simulink model "LAB1_REDES_CONV"  (R2024b)
settings: Solver=VariableStepAuto  StartTime=0.0  StopTime=inf  RelTol=1e-3
undefined symbols (not defined in the file): QAM
libraries: simulink_extras x4, commdigbbndam3 x2, dspvision x1, simulink x1, commrandsrc3 x1
settings Model: Creator=ASUS  LastModifiedBy=ASUS

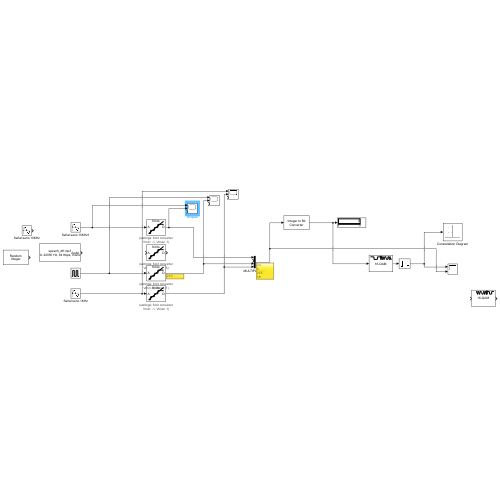
[thumbnail: Simulink's stored preview of the top-level diagram]
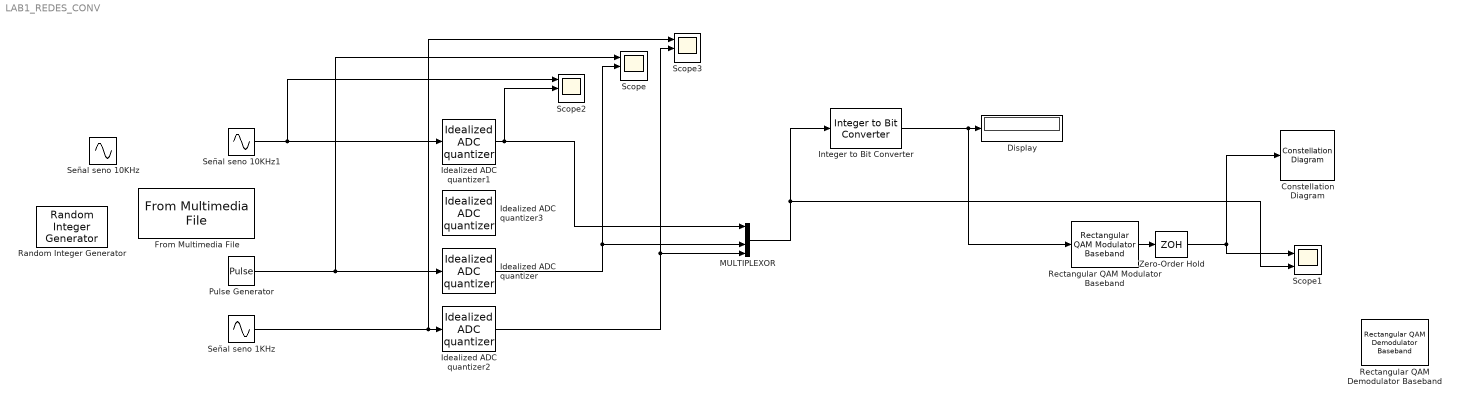
== system LAB1_REDES_CONV ==
  Constellation Diagram : ConstellationDiagram  WindowPosition=[88.000000,123.000000,600.000000,600.000000,]  Visible=on  ScopeFrameLocation=window  ReferenceConstellation=16-QAM  XLimits=[-1.24,1.38]  YLimits=[-1.15,1.28]  ShowReferenceConstellation=off  MeasurementInterval=All displays  DefaultConfigurationName=comm.scopes.ConstellationDiagramBlockCfg
  Display : Display
  From Multimedia File : dspvision/From Multimedia File  inputFilename=speech_dft.mp3  readRange=[1 Inf]  loop=on  numPlays=inf  outputStreams=Audio only  videoDataType=single  audioDataType=double  inheritSampleTime=on  userDefinedSampleTime=1/30  noAudioOutput=off  isIntensityVideo=off  fourcc=RGB  colorVideoFormat=Separate color signals  outputEOF=off  dataOrg=Column-major  audioFrameSize=1024  computeAudioFrameSize=off  outSamplingMode=Sample based
      settings: LibrarySourceBlock=audiosources/From Multimedia File
  Idealized ADC quantizer : simulink_extras/Additional Discrete/Idealized ADC quantizer  NumberOfConverterBits=8  Vmin=0  Vmax=1  OutputDataType=uint8  OutputNegativeValues=on
  Idealized ADC quantizer1 : simulink_extras/Additional Discrete/Idealized ADC quantizer  NumberOfConverterBits=8  Vmin=-1  Vmax=1  OutputDataType=uint8  OutputNegativeValues=off
  Idealized ADC quantizer2 : simulink_extras/Additional Discrete/Idealized ADC quantizer  NumberOfConverterBits=8  Vmin=-1  Vmax=1  OutputDataType=uint8  OutputNegativeValues=off
  Idealized ADC quantizer3 : simulink_extras/Additional Discrete/Idealized ADC quantizer  NumberOfConverterBits=8  Vmin=0  Vmax=5  OutputDataType=uint8  OutputNegativeValues=on
  Integer to Bit Converter : simulink/Logic and Bit Operations/Integer to Bit Converter  nbits=8  signedInputValues=Unsigned  bitOrder=MSB first  outDtype=Inherit via internal rule
  MULTIPLEXOR : Mux
  Pulse Generator : DiscretePulseGenerator  PulseType=Time based  Period=10  PulseWidth=50
  Random Integer Generator : commrandsrc3/Random Integer Generator  SetSize=16  SeedSource=Auto  Seed=0  SampleTime=1  SamplesPerFrame=100  OutputDataType=double  SimulateUsing=Interpreted execution
  Rectangular QAM Demodulator Baseband : commdigbbndam3/Rectangular QAM Demodulator Baseband  M=16  OutType=Integer  DecType=Hard decision  VarSource=Dialog  Variance=1  Dec=Gray  Mapping=[0:15]  PowType=Min. distance between symbols  MinDist=2  AvgPow=1  PeakPow=1  Ph=0  outDtype1=Inherit via internal rule  outDtype2=Inherit via internal rule  derotateFactorWordLen=16  derotateFactorDataTypeStr=Inherit: Same word length as input  derotateFactorLastDataTypeStr=Inherit: Same word length as input  denormFactorWordLen=16  denormFactorDataTypeStr=Inherit: Same word length as input  denormFactorLastDataTypeStr=Inherit: Same word length as input  prodOutWordLen=32  prodOutOverflowMode=Wrap  prodOutRoundingMode=Floor  prodOutOvFlMode=off  prodOutOvFlModeLastStrValue=off  sumWordLen=32
  Rectangular QAM Modulator Baseband : commdigbbndam3/Rectangular QAM Modulator Baseband  M=16  InType=Bit  Enc=Gray  Mapping=[0:15]  PowType=Average Power  MinDist=2  AvgPow=1  PeakPow=1  Ph=0  outDtype=double  outWordLen=16  outUDDataType=sfix(16)  outFracLenMode=Best precision  outFracLen=15  outDataTypeStr=double  outLastDataTypeStr=double
  Scope : Scope  NumInputPorts=3
  Scope1 : Scope  NumInputPorts=2
  Scope2 : Scope  NumInputPorts=3
  Scope3 : Scope  NumInputPorts=3
  Señal seno 10KHz : Sin  Frequency=62832  SampleTime=0
  Señal seno 10KHz1 : Sin  Frequency=100  SampleTime=0
  Señal seno 1KHz : Sin  Frequency=6283  SampleTime=0
  Zero-Order Hold : ZeroOrderHold  SampleTime=0.0001
  wires:
  Pulse Generator/1 -> Idealized ADC quantizer/1, Scope/1
  Señal seno 1KHz/1 -> Scope3/1, Idealized ADC quantizer2/1
  Señal seno 10KHz1/1 -> Scope2/1, Idealized ADC quantizer1/1
  Idealized ADC quantizer1/1 -> Scope2/2, MULTIPLEXOR/1
  Idealized ADC quantizer/1 -> Scope/2, MULTIPLEXOR/3
  Idealized ADC quantizer2/1 -> MULTIPLEXOR/4, Scope3/2
  Rectangular QAM Modulator Baseband/1 -> Zero-Order Hold/1
  MULTIPLEXOR/1 -> Scope1/2, Integer to Bit Converter/1
  Integer to Bit Converter/1 -> Rectangular QAM Modulator Baseband/1, Display/1
  Zero-Order Hold/1 -> Constellation Diagram/1, Scope1/1
